simulink model "kalman_verifier"  (R2013b)
settings: Solver=FixedStepDiscrete  StartTime=0  StopTime=45  FixedStep=0.05  RelTol=1e-3
settings Model: Creator=Franta  LastModifiedBy=Franta

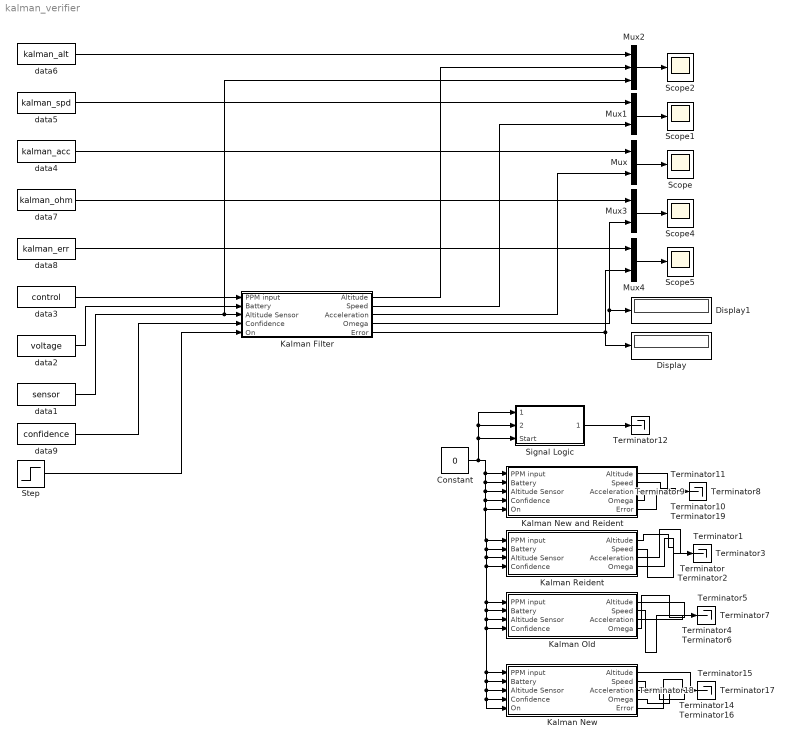
== system kalman_verifier ==
  Constant : Constant  Value=0
  Display : Display
  Display1 : Display
  Kalman Filter : Subsystem
  Kalman New : Subsystem
  Kalman New and Reident : Subsystem
  Kalman Old : Subsystem
  Kalman Reident : Subsystem
  Mux{,1,3..4} (4 alike) : Mux  Inputs=2
  Mux2 : Mux  Inputs=3
  Scope{,1..2,4..5} (5 alike) : Scope
      Scope settings: YMin=0  YMax=47.5
      Scope1 settings: TimeRange=50
      Scope2 settings: SaveName=ScopeData2
      Scope4 settings: YMin=0  YMax=47.5  SaveName=ScopeData4
      Scope5 settings: YMin=0  YMax=47.5  SaveName=ScopeData5
  Signal Logic : Subsystem
  Step : Step  Time=11  SampleTime=0
  Terminator{,1..12,14..19} (19 alike) : Terminator
  data1 : FromWorkspace  VariableName=sensor  SampleTime=0  OutputAfterFinalValue=Holding final value
  data2 : FromWorkspace  VariableName=voltage  SampleTime=0  OutputAfterFinalValue=Holding final value
  data3 : FromWorkspace  VariableName=control  SampleTime=0  OutputAfterFinalValue=Holding final value
  data4 : FromWorkspace  VariableName=kalman_acc  SampleTime=0  OutputAfterFinalValue=Holding final value
  data5 : FromWorkspace  VariableName=kalman_spd  SampleTime=0  OutputAfterFinalValue=Holding final value
  data6 : FromWorkspace  VariableName=kalman_alt  SampleTime=0  OutputAfterFinalValue=Holding final value
  data7 : FromWorkspace  VariableName=kalman_ohm  SampleTime=0  OutputAfterFinalValue=Holding final value
  data8 : FromWorkspace  VariableName=kalman_err  SampleTime=0  OutputAfterFinalValue=Holding final value
  data9 : FromWorkspace  VariableName=confidence  SampleTime=0  OutputAfterFinalValue=Holding final value
  wires:
  Mux/1 -> Scope/1
  Mux1/1 -> Scope1/1
  Mux2/1 -> Scope2/1
  Kalman Filter/3(Acceleration) -> Mux/2
  Kalman Filter/1(Altitude) -> Mux2/2
  Kalman Filter/2(Speed) -> Mux1/2
  Mux3/1 -> Scope4/1
  Mux4/1 -> Scope5/1
  Kalman Filter/5(Error) -> Mux4/2, Display/1
  Kalman Filter/4(Omega) -> Mux3/2, Display1/1
  Kalman Reident/1(Altitude) -> Terminator/1
  Kalman Reident/2(Speed) -> Terminator1/1
  Kalman Reident/3(Acceleration) -> Terminator2/1
  Kalman Reident/4(Omega) -> Terminator3/1
  Kalman Old/1(Altitude) -> Terminator4/1
  Kalman Old/2(Speed) -> Terminator5/1
  Kalman Old/3(Acceleration) -> Terminator6/1
  Kalman Old/4(Omega) -> Terminator7/1
  data1/1 -> Kalman Filter/3(Altitude Sensor), Mux2/3
  data3/1 -> Kalman Filter/1(PPM input)
  data2/1 -> Kalman Filter/2(Battery)
  data5/1 -> Mux1/1
  data4/1 -> Mux/1
  data7/1 -> Mux3/1
  data8/1 -> Mux4/1
  Kalman New and Reident/1(Altitude) -> Terminator8/1
  Kalman New and Reident/2(Speed) -> Terminator9/1
  Kalman New and Reident/3(Acceleration) -> Terminator10/1
  Kalman New and Reident/4(Omega) -> Terminator11/1
  Signal Logic/1(Confidence) -> Terminator12/1
  Kalman New/1(Altitude) -> Terminator14/1
  Kalman New/2(Speed) -> Terminator15/1
  Kalman New/3(Acceleration) -> Terminator16/1
  Kalman New/4(Omega) -> Terminator17/1
  Kalman New/5(Error) -> Terminator18/1
  Kalman New and Reident/5(Error) -> Terminator19/1
  Constant/1 -> Signal Logic/3(Start), Signal Logic/2(Kalman Altitude), Signal Logic/1(Sensor Altitude), Kalman New and Reident/1(PPM input), Kalman New and Reident/2(Battery), Kalman New and Reident/3(Altitude Sensor), Kalman New and Reident/4(Confidence), Kalman New and Reident/5(On), Kalman Reident/4(Confidence), Kalman Old/1(PPM input), Kalman Old/2(Battery), Kalman Old/3(Altitude Sensor), Kalman Old/4(Confidence), Kalman New/1(PPM input), Kalman New/2(Battery), Kalman New/5(On), Kalman New/4(Confidence), Kalman New/3(Altitude Sensor), Kalman Reident/3(Altitude Sensor), Kalman Reident/2(Battery), Kalman Reident/1(PPM input)
  data9/1 -> Kalman Filter/4(Confidence)
  Step/1 -> Kalman Filter/5(On)
  data6/1 -> Mux2/1

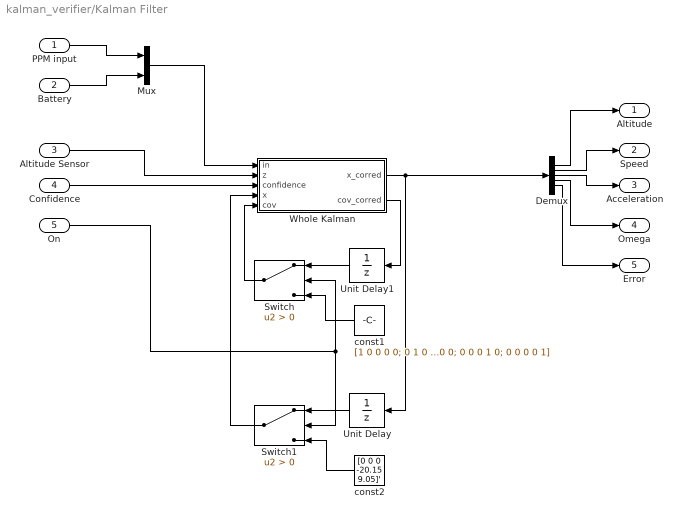
== system kalman_verifier/Kalman Filter ==
  PPM input : Inport
  Battery : Inport  Port=2
  Altitude Sensor : Inport  Port=3
  Confidence : Inport  Port=4
  On : Inport  Port=5
  Demux : Demux  Outputs=5
  Mux : Mux  Inputs=2
  Switch : Switch  Criteria=u2 > Threshold
  Switch1 : Switch  Criteria=u2 > Threshold
  Unit Delay : UnitDelay  InitialCondition=[0 0 0 0 0]'  SampleTime=-1
  Unit Delay1 : UnitDelay  InitialCondition=[1 0 0 0 0; 0 1 0 0 0; 0 0 1 0 0; 0 0 0 1 0; 0 0 0 0 1]  SampleTime=-1
  Whole Kalman : MATLAB Function  TreatAsAtomicUnit=on
  const1 : Constant  Value=[1 0 0 0 0; 0 1 0 0 0; 0 0 1 0 0; 0 0 0 1 0; 0 0 0 0 1]
  const2 : Constant  Value=[0 0 0 -20.15 9.05]'
  Altitude : Outport
  Speed : Outport  Port=2
  Acceleration : Outport  Port=3
  Omega : Outport  Port=4
  Error : Outport  Port=5
  wires:
  Whole Kalman/1(x_corred) -> Demux/1, Unit Delay/1
  Mux/1 -> Whole Kalman/1(in)
  PPM input/1 -> Mux/1
  Battery/1 -> Mux/2
  Demux/2 -> Speed/1
  Demux/3 -> Acceleration/1
  Demux/1 -> Altitude/1
  Demux/4 -> Omega/1
  Whole Kalman/2(cov_corred) -> Unit Delay1/1
  Confidence/1 -> Whole Kalman/3(confidence)
  Altitude Sensor/1 -> Whole Kalman/2(z)
  Unit Delay1/1 -> Switch/1
  Switch/1 -> Whole Kalman/5(cov)
  Unit Delay/1 -> Switch1/1
  Switch1/1 -> Whole Kalman/4(x)
  const1/1 -> Switch/3
  const2/1 -> Switch1/3
  On/1 -> Switch/2, Switch1/2
  Demux/5 -> Error/1

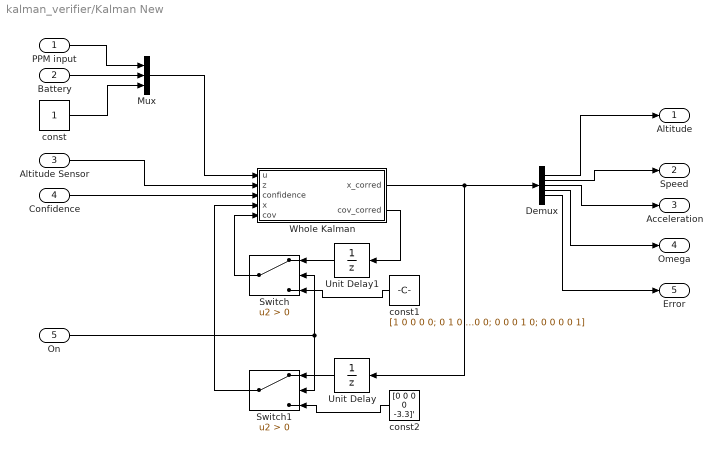
== system kalman_verifier/Kalman New ==
  PPM input : Inport
  Battery : Inport  Port=2
  Altitude Sensor : Inport  Port=3
  Confidence : Inport  Port=4
  On : Inport  Port=5
  Demux : Demux  Outputs=5
  Mux : Mux  Inputs=3
  Switch : Switch  Criteria=u2 > Threshold
  Switch1 : Switch  Criteria=u2 > Threshold
  Unit Delay : UnitDelay  InitialCondition=[0 0 0 0 -10.46]'  SampleTime=-1
  Unit Delay1 : UnitDelay  InitialCondition=[1 0 0 0 0; 0 1 0 0 0; 0 0 1 0 0; 0 0 0 1 0; 0 0 0 0 1]  SampleTime=-1
  Whole Kalman : MATLAB Function  TreatAsAtomicUnit=on
  const : Constant
  const1 : Constant  Value=[1 0 0 0 0; 0 1 0 0 0; 0 0 1 0 0; 0 0 0 1 0; 0 0 0 0 1]
  const2 : Constant  Value=[0 0 0 0 -3.3]'
  Altitude : Outport
  Speed : Outport  Port=2
  Acceleration : Outport  Port=3
  Omega : Outport  Port=4
  Error : Outport  Port=5
  wires:
  On/1 -> Switch1/2, Switch/2
  Demux/1 -> Altitude/1
  Whole Kalman/1(x_corred) -> Demux/1, Unit Delay/1
  const2/1 -> Switch1/3
  const1/1 -> Switch/3
  Switch1/1 -> Whole Kalman/4(x)
  Unit Delay/1 -> Switch1/1
  Switch/1 -> Whole Kalman/5(cov)
  Unit Delay1/1 -> Switch/1
  Altitude Sensor/1 -> Whole Kalman/2(z)
  Confidence/1 -> Whole Kalman/3(confidence)
  Whole Kalman/2(cov_corred) -> Unit Delay1/1
  Demux/4 -> Omega/1
  Demux/3 -> Acceleration/1
  Demux/2 -> Speed/1
  const/1 -> Mux/3
  Battery/1 -> Mux/2
  PPM input/1 -> Mux/1
  Mux/1 -> Whole Kalman/1(u)
  Demux/5 -> Error/1

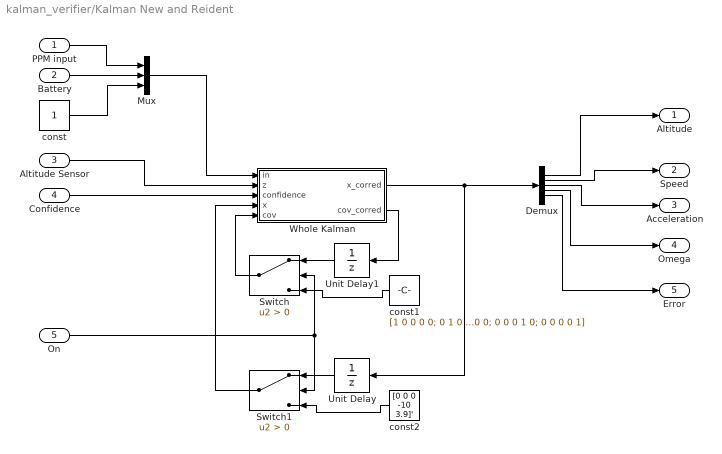
== system kalman_verifier/Kalman New and Reident ==
  PPM input : Inport
  Battery : Inport  Port=2
  Altitude Sensor : Inport  Port=3
  Confidence : Inport  Port=4
  On : Inport  Port=5
  Demux : Demux  Outputs=5
  Mux : Mux  Inputs=3
  Switch : Switch  Criteria=u2 > Threshold
  Switch1 : Switch  Criteria=u2 > Threshold
  Unit Delay : UnitDelay  InitialCondition=[0 0 0 0 -10.46]'  SampleTime=-1
  Unit Delay1 : UnitDelay  InitialCondition=[1 0 0 0 0; 0 1 0 0 0; 0 0 1 0 0; 0 0 0 1 0; 0 0 0 0 1]  SampleTime=-1
  Whole Kalman : MATLAB Function  TreatAsAtomicUnit=on
  const : Constant
  const1 : Constant  Value=[1 0 0 0 0; 0 1 0 0 0; 0 0 1 0 0; 0 0 0 1 0; 0 0 0 0 1]
  const2 : Constant  Value=[0 0 0 -10 3.9]'
  Altitude : Outport
  Speed : Outport  Port=2
  Acceleration : Outport  Port=3
  Omega : Outport  Port=4
  Error : Outport  Port=5
  wires:
  Demux/5 -> Error/1
  Mux/1 -> Whole Kalman/1(in)
  PPM input/1 -> Mux/1
  Battery/1 -> Mux/2
  const/1 -> Mux/3
  Demux/2 -> Speed/1
  Demux/3 -> Acceleration/1
  Demux/4 -> Omega/1
  Whole Kalman/2(cov_corred) -> Unit Delay1/1
  Confidence/1 -> Whole Kalman/3(confidence)
  Altitude Sensor/1 -> Whole Kalman/2(z)
  Unit Delay1/1 -> Switch/1
  Switch/1 -> Whole Kalman/5(cov)
  Unit Delay/1 -> Switch1/1
  Switch1/1 -> Whole Kalman/4(x)
  const1/1 -> Switch/3
  const2/1 -> Switch1/3
  Whole Kalman/1(x_corred) -> Unit Delay/1, Demux/1
  Demux/1 -> Altitude/1
  On/1 -> Switch/2, Switch1/2

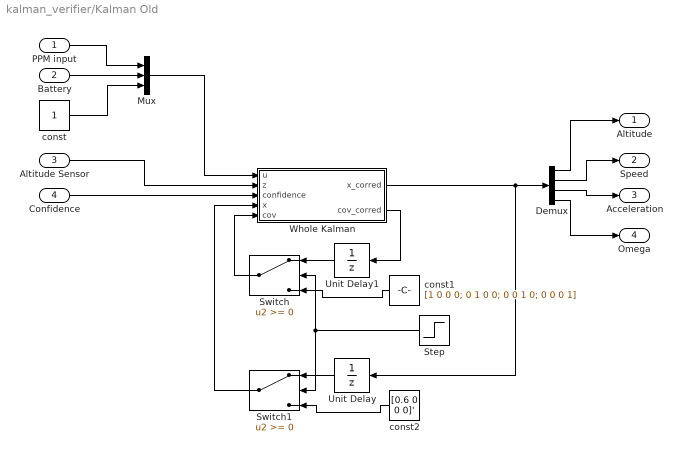
== system kalman_verifier/Kalman Old ==
  PPM input : Inport
  Battery : Inport  Port=2
  Altitude Sensor : Inport  Port=3
  Confidence : Inport  Port=4
  Demux : Demux
  Mux : Mux  Inputs=3
  Step : Step  Time=7.5  Before=-1  SampleTime=0
  Switch : Switch
  Switch1 : Switch
  Unit Delay : UnitDelay  InitialCondition=[0.6 0 0 0]'  SampleTime=-1
  Unit Delay1 : UnitDelay  InitialCondition=[1 0 0 0; 0 1 0 0; 0 0 1 0; 0 0 0 1]  SampleTime=-1
  Whole Kalman : MATLAB Function  TreatAsAtomicUnit=on
  const : Constant
  const1 : Constant  Value=[1 0 0 0; 0 1 0 0; 0 0 1 0; 0 0 0 1]
  const2 : Constant  Value=[0.6 0 0 0]'
  Altitude : Outport
  Speed : Outport  Port=2
  Acceleration : Outport  Port=3
  Omega : Outport  Port=4
  wires:
  Whole Kalman/1(x_corred) -> Demux/1, Unit Delay/1
  Mux/1 -> Whole Kalman/1(u)
  PPM input/1 -> Mux/1
  Battery/1 -> Mux/2
  const/1 -> Mux/3
  Demux/2 -> Speed/1
  Demux/3 -> Acceleration/1
  Demux/1 -> Altitude/1
  Demux/4 -> Omega/1
  Whole Kalman/2(cov_corred) -> Unit Delay1/1
  Confidence/1 -> Whole Kalman/3(confidence)
  Altitude Sensor/1 -> Whole Kalman/2(z)
  Unit Delay1/1 -> Switch/1
  Switch/1 -> Whole Kalman/5(cov)
  Unit Delay/1 -> Switch1/1
  Switch1/1 -> Whole Kalman/4(x)
  Step/1 -> Switch1/2, Switch/2
  const1/1 -> Switch/3
  const2/1 -> Switch1/3

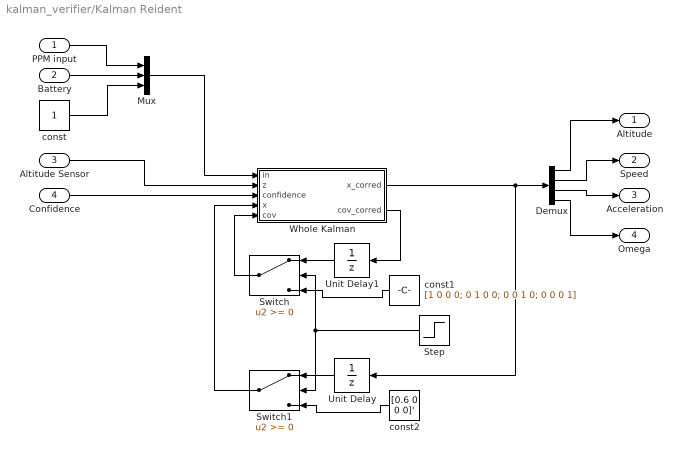
== system kalman_verifier/Kalman Reident ==
  PPM input : Inport
  Battery : Inport  Port=2
  Altitude Sensor : Inport  Port=3
  Confidence : Inport  Port=4
  Demux : Demux
  Mux : Mux  Inputs=3
  Step : Step  Time=7.5  Before=-1  SampleTime=0
  Switch : Switch
  Switch1 : Switch
  Unit Delay : UnitDelay  InitialCondition=[0.6 0 0 0]'  SampleTime=-1
  Unit Delay1 : UnitDelay  InitialCondition=[1 0 0 0; 0 1 0 0; 0 0 1 0; 0 0 0 1]  SampleTime=-1
  Whole Kalman : MATLAB Function  TreatAsAtomicUnit=on
  const : Constant
  const1 : Constant  Value=[1 0 0 0; 0 1 0 0; 0 0 1 0; 0 0 0 1]
  const2 : Constant  Value=[0.6 0 0 0]'
  Altitude : Outport
  Speed : Outport  Port=2
  Acceleration : Outport  Port=3
  Omega : Outport  Port=4
  wires:
  const2/1 -> Switch1/3
  const1/1 -> Switch/3
  Step/1 -> Switch/2, Switch1/2
  Switch1/1 -> Whole Kalman/4(x)
  Unit Delay/1 -> Switch1/1
  Switch/1 -> Whole Kalman/5(cov)
  Unit Delay1/1 -> Switch/1
  Altitude Sensor/1 -> Whole Kalman/2(z)
  Confidence/1 -> Whole Kalman/3(confidence)
  Whole Kalman/2(cov_corred) -> Unit Delay1/1
  Demux/4 -> Omega/1
  Demux/1 -> Altitude/1
  Demux/3 -> Acceleration/1
  Demux/2 -> Speed/1
  const/1 -> Mux/3
  Battery/1 -> Mux/2
  PPM input/1 -> Mux/1
  Mux/1 -> Whole Kalman/1(in)
  Whole Kalman/1(x_corred) -> Unit Delay/1, Demux/1

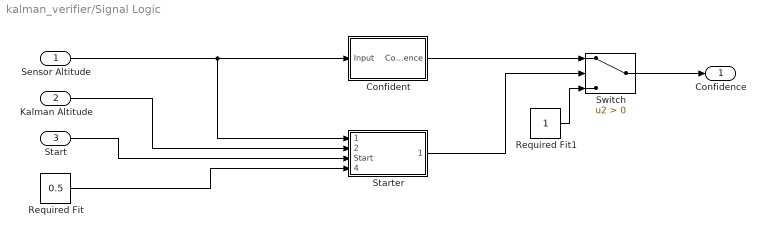
== system kalman_verifier/Signal Logic ==
  Sensor Altitude : Inport
  Kalman Altitude : Inport  Port=2
  Start : Inport  Port=3
  Confident : Subsystem
  Required Fit : Constant  Value=0.5
  Required Fit1 : Constant
  Starter : Subsystem
  Switch : Switch  Criteria=u2 > Threshold
  Confidence : Outport
  wires:
  Sensor Altitude/1 -> Starter/1(Sensor Altitude), Confident/1(Input)
  Start/1 -> Starter/3(Start)
  Switch/1 -> Confidence/1
  Required Fit/1 -> Starter/4(Required Fit)
  Kalman Altitude/1 -> Starter/2(Kalman Altitude)
  Confident/1(Confidence) -> Switch/1
  Starter/1(Confidence Override) -> Switch/2
  Required Fit1/1 -> Switch/3

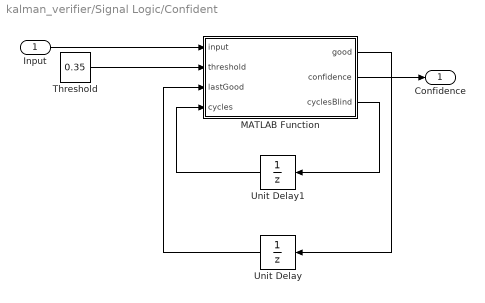
== system kalman_verifier/Signal Logic/Confident ==
  Input : Inport
  MATLAB Function : MATLAB Function  TreatAsAtomicUnit=on
  Threshold : Constant  Value=0.35
  Unit Delay : UnitDelay  InitialCondition=0.5  SampleTime=-1
  Unit Delay1 : UnitDelay  SampleTime=-1
  Confidence : Outport
  wires:
  Input/1 -> MATLAB Function/1(input)
  Threshold/1 -> MATLAB Function/2(threshold)
  MATLAB Function/1(good) -> Unit Delay/1
  Unit Delay/1 -> MATLAB Function/3(lastGood)
  MATLAB Function/2(confidence) -> Confidence/1
  MATLAB Function/3(cyclesBlind) -> Unit Delay1/1
  Unit Delay1/1 -> MATLAB Function/4(cycles)

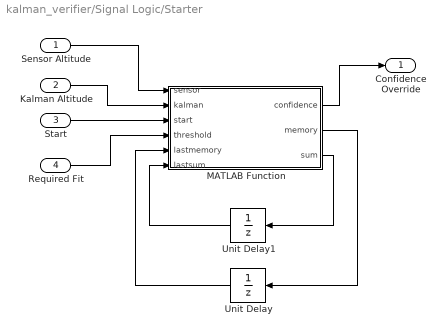
== system kalman_verifier/Signal Logic/Starter ==
  Sensor Altitude : Inport
  Kalman Altitude : Inport  Port=2
  Start : Inport  Port=3
  Required Fit : Inport  Port=4
  MATLAB Function : MATLAB Function  TreatAsAtomicUnit=on
  Unit Delay : UnitDelay  InitialCondition="[0 0 0 0 0 0 0 0 0 0  0 0 0 0 0 0 0 0 0 0]"  SampleTime=-1
  Unit Delay1 : UnitDelay  SampleTime=-1
  Confidence Override : Outport
  wires:
  Sensor Altitude/1 -> MATLAB Function/1(sensor)
  Start/1 -> MATLAB Function/3(start)
  MATLAB Function/1(confidence) -> Confidence Override/1
  Unit Delay/1 -> MATLAB Function/5(lastmemory)
  Required Fit/1 -> MATLAB Function/4(threshold)
  Kalman Altitude/1 -> MATLAB Function/2(kalman)
  MATLAB Function/2(memory) -> Unit Delay/1
  MATLAB Function/3(sum) -> Unit Delay1/1
  Unit Delay1/1 -> MATLAB Function/6(lastsum)

== matlab function kalman_verifier/Kalman Old/Whole Kalman ==
  data: u input; z input; confidence input; x_corred output; cov_corred output; x input; cov input
function [x_corred, cov_corred] = kalman(u, z, confidence, x, cov)
A = [1 0.05 0 0; 0 1 0.05 0; 0 0 0 1; 0 0 -0.65658 1.5714];
B = [0 0 0; 0 0 0; 0.00091141 -0.36830 -2.8005; 0.0011525 -0.052414 -7.5757];
P = [1 0 0 0];
Q = 1/confidence;
R = [1 0 0 0; 0 1 0 0; 0 0 1 0; 0 0 0 1];

%prediction
x_next = A*x + B*u;
cov_next = (A*cov*A') + R;

%correction
if (confidence > 0.001)
    K = (cov_next*P')/((P*cov_next*P') + Q);
    x_corred = x_next + K*(z - P*x_next);
    cov_corred = (eye(4) - K*P)*cov_next;
else
    x_corred = x_next;
    cov_corred = cov_next;
end

== matlab function kalman_verifier/Kalman Reident/Whole Kalman ==
  data: in input; z input; confidence input; x_corred output; cov_corred output; x input; cov input
function [x_corred, cov_corred] = kalman(in, z, confidence, x, cov)
u = ((in(1)/100) + (in(2)*2.3) -91.65);
A = [1 0.05 0 0; 0 1 0.05 0; 0 0 0 1; 0 0 -0.742912189150098 1.679723128361149];
B = [0; 0; 0.104540214230006; 0.111455526107170];
P = [1 0 0 0];
Q = 100/confidence;
R = [1 0 0 0; 0 1 0 0; 0 0 1 0; 0 0 0 1];

%prediction
x_next = A*x + B*u;
cov_next = (A*cov*A') + R;

%correction
if (confidence > 0.001)
    K = (cov_next*P')/((P*cov_next*P') + Q);
    x_corred = x_next + K*(z - P*x_next);
    cov_corred = (eye(4) - K*P)*cov_next;
else
    x_corred = x_next;
    cov_corred = cov_next;
end

== matlab function kalman_verifier/Kalman New/Whole Kalman ==
  data: u input; z input; confidence input; x_corred output; cov_corred output; x input; cov input
function [x_corred, cov_corred] = kalman(u, z, confidence, x, cov)
A = [1 0.05 0 0 0; 0 1 0.05 0 0; 0 0 0 1 1; 0 0 -0.65658 1.5714 0; 0 0 0 0 1];
B = [0 0 0; 0 0 0; 0.00091141 -0.36830 -2.8005; 0.0011525 -0.052414 -7.5757; 0 0 0];
P = [1 0 0 0 0];
Q = 100/confidence;
R = [1 0 0 0 0; 0 1 0 0 0; 0 0 1 0 0; 0 0 0 1 0; 0 0 0 0 1];

%prediction
x_next = A*x + B*u;
cov_next = (A*cov*A') + R;

%correction
if (confidence > 0.001)
    K = (cov_next*P')/((P*cov_next*P') + Q);
    x_corred = x_next + K*(z - P*x_next);
    cov_corred = (eye(5) - K*P)*cov_next;
else
    x_corred = x_next;
    cov_corred = cov_next;
end

== matlab function kalman_verifier/Kalman Filter/Whole Kalman ==
  data: in input; z input; confidence input; x_corred output; cov_corred output; x input; cov input
function [x_corred, cov_corred] = kalman(in, z, confidence, x, cov)
u = ((in(1)/100) + (in(2)*2.3));
A = [1 0.05 0 0 0; 0 1 0.05 0 0; 0 0 0 1 1; 0 0 -0.66953 1.58995 0; 0 0 0 0 1];
B = [0; 0; 0.11700; 0.12710; 0];
P = [1 0 0 0 0];
Q = 100/confidence;
R = [1 0 0 0 0; 0 1 0 0 0; 0 0 1 0 0; 0 0 0 1 0; 0 0 0 0 1];

% prediction
x_next = A*x + B*u;
cov_next = (A*cov*A') + R;

% correction
if (confidence > 0.001)
    K = (cov_next*P')/((P*cov_next*P') + Q);
    x_corred = x_next + K*(z - P*x_next);
    cov_corred = (eye(5) - K*P)*cov_next;
else % do not correct
    x_corred = x_next;
    cov_corred = cov_next;
end

== matlab function kalman_verifier/Kalman New and Reident/Whole Kalman ==
  data: in input; z input; confidence input; x_corred output; cov_corred output; x input; cov input
function [x_corred, cov_corred] = kalman(in, z, confidence, x, cov)
u = ((in(1)/100) + (in(2)*2.3));
A = [1 0.05 0 0 0; 0 1 0.05 0 0; 0 0 0 1 1; 0 0 -0.74291 1.67972 0; 0 0 0 0 1];
B = [0; 0; 0.10454; 0.11146; 0];
P = [1 0 0 0 0];
Q = 100/confidence;
R = [1 0 0 0 0; 0 1 0 0 0; 0 0 1 0 0; 0 0 0 1 0; 0 0 0 0 1];

%prediction
x_next = A*x + B*u;
cov_next = (A*cov*A') + R;

%correction
if (confidence > 0.001)
    K = (cov_next*P')/((P*cov_next*P') + Q);
    x_corred = x_next + K*(z - P*x_next);
    cov_corred = (eye(5) - K*P)*cov_next;
else
    x_corred = x_next;
    cov_corred = cov_next;
end

== matlab function kalman_verifier/Signal Logic/Confident/MATLAB Function ==
  data: input input; threshold input; good output; lastGood input; confidence output; cycles input; cyclesBlind output
function [good, confidence, cyclesBlind] = confident(input, threshold, lastGood, cycles)

if (input == lastGood)
        if (cycles < 16)
            good = lastGood;    
            confidence = 1 - (cycles/16)^2;
            cyclesBlind = cycles + 1;
        else
            good = lastGood;  
            confidence = 0;
            cyclesBlind = cycles + 1;
        end     
else
    if (abs(input - lastGood) > threshold)
        if (cycles < 16)
            good = lastGood;
            confidence = (2^cycles)/65536;
            cyclesBlind = cycles + 1;
        else
            good = input;
            confidence = 1;
            cyclesBlind = 0;
        end        
    else
        good = input;
        confidence = 1;
        cyclesBlind = 0;
    end
end

== matlab function kalman_verifier/Signal Logic/Starter/MATLAB Function ==
  data: confidence output; sensor input; kalman input; start input; threshold input; lastmemory input; lastsum input; memory output; sum output
function [confidence, memory, sum] = starter(sensor, kalman, start, threshold, lastmemory, lastsum)

if (start > 0)
    memory = zeros(20, 1);
    memory(1) = abs(sensor - kalman);
    memory(2:20) = lastmemory(1:19);
    sum = lastsum - lastmemory(20) + memory(1);
        if (lastsum > threshold)
            confidence = 1;
        else
            confidence = 0;
        end     
else
    sum = 2;
    memory = 0.1*ones(20, 1);
    confidence = 1;
end
